simulink model "ATRIAS_vnmc"  (R2015a)
settings: Solver=ode45  StartTime=0.0  StopTime=60  FixedStep=1e-3  MinStep=1e-6  RelTol=1e-3  AbsTol=1e-4
values from neighbouring files (symbols this model uses):
  initial_boom_yaw = initial_boom_yaw + delta_yaw0    [run_model.m]
  max_floor_diff = cost_fun_opts.max_floor_diff    [opt_cmaes.m]    (also in run_model.m; set_all_params_simple.m = 0)
  noise_on_off = cost_fun_opts.noise_on_off    [opt_cmaes.m]    (also in run_model.m; set_all_params_simple.m = 0)
  noise_seed = cost_fun_opts.noise_seed    [opt_cmaes.m]    (also in run_model.m; set_all_params_simple.m = 1)
  noise_variance = cost_fun_opts.noise_variance    [opt_cmaes.m]    (also in run_model.m; set_all_params_simple.m = 0.000174532925199)
  SEA_swing_ctrl_on_off = cost_fun_opts.SEA_swing_ctrl_on_off    [opt_cmaes.m]    (also in run_model.m; set_all_params_simple.m = 0)
  sim_t = simout.twalk    [run_model.m]
  steady_dist = cost_fun_opts.steady_dist    [opt_cmaes.m]    (also in run_model.m; set_all_params_simple.m = 10)
  ts_anim = 0.0333    [run_model.m]
undefined symbols (not defined in the file or in its folder): A1_notch_f1, A2_notch_f1, A_lpf_dtau, A_lpf_velocity, B1_lpf_dtau, B1_lpf_velocity, B1_notch_f1, B2_lpf_dtau, B2_lpf_velocity, B2_notch_f1, b_hmotor, b_leg_spring, b_rotor, base_color_d, boom_color_d, boom_mount_to_center_diagonal, breakaway_friction, c, c_jointstop, com_height_offset, contactThr, coulomb_friction, CtrlPar_theta0, D12_S, D12_T, d_com, ddx_max, ddy_max, delta_phi_max, delta_phi_max_buffer, delta_phi_max_dropoff, delta_phi_min, des_forward_velocity, DS_width, dtau_des_max, dtheta0_vmc, dx0_vmc, dy_max, eref, fblink_color_d, fcut_acceleration, floor_color_d, floor_tile_width, floor_zero_height, FmaxBFSH, FmaxGLU, FmaxHAM, FmaxHFL, FmaxRF, FmaxVAS, FPCtrlPar, friction_linear_zone, g, gain_nodes_sea_torque, gamma_stance_thr, gamma_swing_thr, hip_height, HIP_MTR_MAX_CONT_TORQUE, HIP_MTR_MAX_TORQUE, hshaft_color_d ... (+236)
libraries: sm_lib x280, nesl_utility x174, simulink x114, simulink_extras x58, fl_lib x16, mblibv1 x2, dspswit3 x2
(part 7 of 23)

== system ATRIAS_vnmc/control/Add Limit Avoidance PD Torques/dtau_des ==
  x : Inport
  Gain1 : Gain  Gain=1/sample_time
  difference : simulink/Discrete/Difference  ICPrevInput=0.0  InputProcessing=Inherited  OutMin=[]  OutMax=[]  OutDataType=fixdt(1, 16)  OutScaling=2^-10  DoSatur=off
  two_pole_filter : DiscreteTransferFcn  Numerator=[A_lpf_dtau 0 0]  Denominator=[1 B1_lpf_dtau B2_lpf_dtau]  SampleTime=sample_time
  dx/dt : Outport
  wires:
  two_pole_filter/1 -> dx/dt/1
  x/1 -> Gain1/1
  difference/1 -> two_pole_filter/1
  Gain1/1 -> difference/1

== system ATRIAS_vnmc/control/Add Limit Avoidance PD Torques/mechanical limit avoidance ==
  tau_des [Nm]x4 : Inport
  PD Joint Limit : Subsystem
  Product : Product
  Sum : Sum  Inputs=++|
  tau_des + pd [Nm]x4 : Outport
  wires:
  tau_des [Nm]x4/1 -> Product/2
  PD Joint Limit/1(tau_pd [Nm]x4) -> Sum/1
  Sum/1 -> tau_des + pd [Nm]x4/1
  PD Joint Limit/2(des_trq_scale x4) -> Product/1
  Product/1 -> Sum/2

== system ATRIAS_vnmc/control/Export Results/Contact and GRFs ==
  note: BASED ON Leg Load
  note: BASED ON Foot Height
  Data Type Conversion{1..3,12} (4 alike) : DataTypeConversion  OutDataTypeStr=double
  Mux1 : Mux  Inputs=2
  Mux2 : Mux  Inputs=2
  Mux3 : Mux  Inputs=3
  Mux4 : Mux  Inputs=2
  10 : Outport
  wires:
  [RHeelCont] -> Data Type Conversion12/1
  [LHeelCont] -> Data Type Conversion1/1
  Mux3/1 -> 10/1
  Mux1/1 -> Mux3/1  "2"
  Data Type Conversion12/1 -> Mux1/1
  Data Type Conversion1/1 -> Mux1/2
  [RHeel_GRF] -> Mux2/1
  Mux2/1 -> Mux3/3  "2x3"
  [LHeel_GRF] -> Mux2/2
  [RFootCnt] -> Data Type Conversion3/1
  [LFootCnt] -> Data Type Conversion2/1
  Data Type Conversion3/1 -> Mux4/1
  Data Type Conversion2/1 -> Mux4/2
  Mux4/1 -> Mux3/2  "2"

== system ATRIAS_vnmc/control/Export Results/Segment Kinematics (position, orientation) ==
  Mux1 : Mux  Inputs=14
  Mux2 : Mux  Inputs=14
  Mux6 : Mux  Inputs=2
  98 : Outport
  wires:
  [xyzBoomBase] -> Mux1/1
  [xyzYawShaft] -> Mux1/2
  [xyzBoom] -> Mux1/3
  [xyzTorso] -> Mux1/4
  [RxyzHipShaft] -> Mux1/5
  [RxyzThigh] -> Mux1/6
  [RxyzShin] -> Mux1/7
  [RxyzLowerLeg] -> Mux1/8
  [RxyzFBlink] -> Mux1/9
  [LxyzLowerLeg] -> Mux1/13
  [LxyzFBlink] -> Mux1/14
  [LxyzHipShaft] -> Mux1/10
  [LxyzThigh] -> Mux1/11
  [LxyzShin] -> Mux1/12
  Mux1/1 -> Mux6/1  "position 42 = 14x3"
  [QBoomBase] -> Mux2/1
  [QYawShaft] -> Mux2/2
  [QBoom] -> Mux2/3
  [QTorso] -> Mux2/4
  [RQHipShaft] -> Mux2/5
  [RQThigh] -> Mux2/6
  [RQShin] -> Mux2/7
  [RQLowerLeg] -> Mux2/8
  [RQFBlink] -> Mux2/9
  [LQHipShaft] -> Mux2/10
  [LQThigh] -> Mux2/11
  [LQShin] -> Mux2/12
  [LQLowerLeg] -> Mux2/13
  [LQFBlink] -> Mux2/14
  Mux2/1 -> Mux6/2  "orientaion 56 = 14x4"
  Mux6/1 -> 98/1

== system ATRIAS_vnmc/control/Export Results/alpha targets ==
  Mux19 : Mux  Inputs=2
  2 : Outport
  wires:
  Mux19/1 -> 2/1
  [Ralpha_tgt] -> Mux19/1
  [Lalpha_tgt] -> Mux19/2

== system ATRIAS_vnmc/control/Export Results/track yaw ==
  xz : Inport
  Abs : Abs
  Compare To Constant : simulink/Logic and Bit Operations/Compare To Constant  relop=>  const=pi  OutDataTypeStr=boolean
  Gain : Gain  Gain=180/pi
  Gain1 : Gain  Gain=180/pi
  Gain2 : Gain  Gain=180/pi
  Memory : Memory
  Scope : Scope  NumInputPorts=4
      settings: YMin=-5~-5~-5~-5  YMax=5~5~5~5
  Sign : Signum
  Sum1 : Sum  Inputs=++|
  Sum2 : Sum  Inputs=|-+
  n*2*pi : Subsystem  TreatAsAtomicUnit=on
  "xz_to_yaw ([0, 2*pi])" : Fcn  Expr=atan2(u(1),-u(2)) +2*pi*(atan2(u(1),-u(2))<0)
  yaw : Outport
  wires:
  Sign/1 -> n*2*pi/2(sign)
  xz/1 -> "xz_to_yaw ([0, 2*pi])"/1
  "xz_to_yaw ([0, 2*pi])"/1 -> Memory/1, Gain1/1, Sum1/2, Sum2/2
  n*2*pi/1(n*2*pi) -> Gain/1, n*2*pi/1((n-1)*2*pi), Sum1/1
  Sum2/1 -> Sign/1, Abs/1
  Abs/1 -> Gain2/1, Compare To Constant/1
  Memory/1 -> Sum2/1
  Compare To Constant/1 -> Scope/3, n*2*pi/Trigger
  Sum1/1 -> yaw/1
  Gain/1 -> Scope/1
  Gain1/1 -> Scope/2
  Gain2/1 -> Scope/4

== system ATRIAS_vnmc/control/Monitor Simulation/Check Ground Penetration ==
  xyz : Inport
  Ground H : Interpolation_n-D  NumberOfTableDimensions=1  Table=v_plateH
      settings: InputPortMap=u0,u1
  Prelookup : PreLookup  BreakpointsData=v_plateYaw  ExtrapMethod=Linear
  Relational Operator : RelationalOperator  Operator=<=  OutDataTypeStr=boolean
  Selector1 : Selector  InputPortWidth=3  Indices=[1 3]
  Selector2 : Selector  InputPortWidth=3  Indices=2
  track yaw : Subsystem
  Below Ground : Outport
  wires:
  Prelookup/2 -> Ground H/2
  track yaw/1(yaw) -> Prelookup/1
  Prelookup/1 -> Ground H/1
  Selector1/1 -> track yaw/1(xz)
  Relational Operator/1 -> Below Ground/1
  Selector2/1 -> Relational Operator/1
  xyz/1 -> Selector1/1, Selector2/1
  Ground H/1 -> Relational Operator/2

== system ATRIAS_vnmc/control/Monitor Simulation/Check Ground Penetration1 ==
  xyz : Inport
  Ground H : Interpolation_n-D  NumberOfTableDimensions=1  Table=v_plateH
      settings: InputPortMap=u0,u1
  Prelookup : PreLookup  BreakpointsData=v_plateYaw  ExtrapMethod=Linear
  Relational Operator : RelationalOperator  Operator=<=  OutDataTypeStr=boolean
  Selector1 : Selector  InputPortWidth=3  Indices=[1 3]
  Selector2 : Selector  InputPortWidth=3  Indices=2
  track yaw : Subsystem
  Below Ground : Outport
  wires:
  Prelookup/2 -> Ground H/2
  track yaw/1(yaw) -> Prelookup/1
  Prelookup/1 -> Ground H/1
  Selector1/1 -> track yaw/1(xz)
  Relational Operator/1 -> Below Ground/1
  Selector2/1 -> Relational Operator/1
  xyz/1 -> Selector1/1, Selector2/1
  Ground H/1 -> Relational Operator/2

== system ATRIAS_vnmc/control/Monitor Simulation/Check Ground Penetration2 ==
  xyz : Inport
  Ground H : Interpolation_n-D  NumberOfTableDimensions=1  Table=v_plateH
      settings: InputPortMap=u0,u1
  Prelookup : PreLookup  BreakpointsData=v_plateYaw  ExtrapMethod=Linear
  Relational Operator : RelationalOperator  Operator=<=  OutDataTypeStr=boolean
  Selector1 : Selector  InputPortWidth=3  Indices=[1 3]
  Selector2 : Selector  InputPortWidth=3  Indices=2
  track yaw : Subsystem
  Below Ground : Outport
  wires:
  Prelookup/2 -> Ground H/2
  track yaw/1(yaw) -> Prelookup/1
  Prelookup/1 -> Ground H/1
  Selector1/1 -> track yaw/1(xz)
  Relational Operator/1 -> Below Ground/1
  Selector2/1 -> Relational Operator/1
  xyz/1 -> Selector1/1, Selector2/1
  Ground H/1 -> Relational Operator/2

== system ATRIAS_vnmc/control/Monitor Simulation/Check Ground Penetration3 ==
  xyz : Inport
  Ground H : Interpolation_n-D  NumberOfTableDimensions=1  Table=v_plateH
      settings: InputPortMap=u0,u1
  Prelookup : PreLookup  BreakpointsData=v_plateYaw  ExtrapMethod=Linear
  Relational Operator : RelationalOperator  Operator=<=  OutDataTypeStr=boolean
  Selector1 : Selector  InputPortWidth=3  Indices=[1 3]
  Selector2 : Selector  InputPortWidth=3  Indices=2
  track yaw : Subsystem
  Below Ground : Outport
  wires:
  Prelookup/2 -> Ground H/2
  track yaw/1(yaw) -> Prelookup/1
  Prelookup/1 -> Ground H/1
  Selector1/1 -> track yaw/1(xz)
  Relational Operator/1 -> Below Ground/1
  Selector2/1 -> Relational Operator/1
  xyz/1 -> Selector1/1, Selector2/1
  Ground H/1 -> Relational Operator/2

== system ATRIAS_vnmc/control/Monitor Simulation/Step Length History ==
  footstrike : Inport
  Lx_Heel : Inport  Port=2
  LHeelCont : Inport  Port=3
  RHeelCont : Inport  Port=4
  RxHeel : Inport  Port=5
  Measure Step Length : Subsystem  TreatAsAtomicUnit=on
  Memory1 : Memory
  Queue1 : Subsystem
  x_footstrike : Subsystem
  step length hist : Outport
  wires:
  Lx_Heel/1 -> x_footstrike/2(x_LFoot [m])
  x_footstrike/1(x_footstrike [m]) -> Measure Step Length/2(x_heelstrike [m]), Memory1/1
  LHeelCont/1 -> x_footstrike/3(LHeel Contact [1/0])
  Memory1/1 -> Measure Step Length/1(x_heelstrike_prev [m])
  Measure Step Length/1(Step Length [m]) -> Queue1/2(stepLength0 [m])
  Queue1/1(footLengthHist [m,m,m,m,m,m,m]) -> step length hist/1
  RxHeel/1 -> x_footstrike/5(x_RFoot [m])
  RHeelCont/1 -> x_footstrike/4(RHeel Contact [1/0])
  footstrike/1 -> Queue1/1(footStrike [1/0]), Measure Step Length/Trigger, x_footstrike/1(Footstrike [1/0])

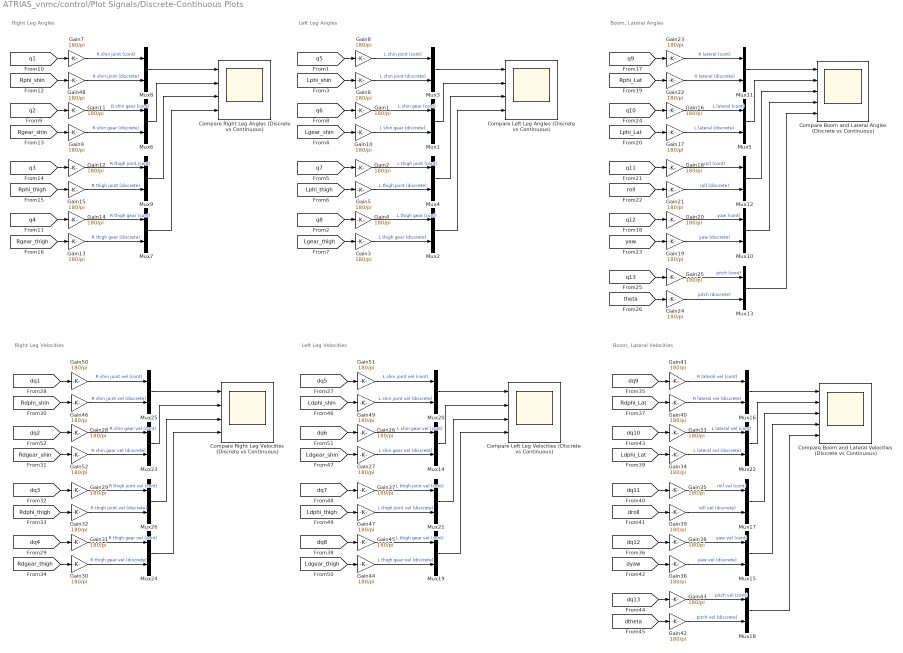
== system ATRIAS_vnmc/control/Plot Signals/Discrete-Continuous Plots ==
  note: Right Leg Angles
  note: Left Leg Angles
  note: Boom, Lateral Angles
  note: Right Leg Velocities
  note: Left Leg Velocities
  note: Boom, Lateral Velocities
  Compare Boom and Lateral Angles (Discrete vs Continuous) : Scope  NumInputPorts=5
      settings: ShowLegends=on  TimeRange=0.895  YMin=152~225.5~132~205.5~-5  YMax=154.5~228~134.5~208~5  SaveName=ScopeData12
  Compare Boom and Lateral Velocities (Discrete vs Continuous) : Scope  NumInputPorts=5
      settings: ShowLegends=on  TimeRange=0.895  YMin=152~225.5~132~205.5~-5  YMax=154.5~228~134.5~208~5  SaveName=ScopeData13
  Compare Left Leg Angles (Discrete vs Continuous) : Scope  NumInputPorts=4
      settings: ShowLegends=on  TimeRange=0.895  YMin=152~225.5~132~205.5  YMax=154.5~228~134.5~208  SaveName=ScopeData11
  Compare Left Leg Velocities (Discrete vs Continuous) : Scope  NumInputPorts=4
      settings: ShowLegends=on  TimeRange=0.895  YMin=152~225.5~132~205.5  YMax=154.5~228~134.5~208  SaveName=ScopeData14
  Compare Right Leg Angles (Discrete vs Continuous) : Scope  NumInputPorts=4
      settings: ShowLegends=on  TimeRange=0.895  YMin=152~225.5~132~205.5  YMax=154.5~228~134.5~208  SaveName=ScopeData8
  Compare Right Leg Velocities (Discrete vs Continuous) : Scope  NumInputPorts=4
      settings: ShowLegends=on  TimeRange=0.895  YMin=152~225.5~132~205.5  YMax=154.5~228~134.5~208  SaveName=ScopeData15
  Gain{1..52} (52 alike) : Gain  Gain=180/pi
  Mux{1..26} (26 alike) : Mux  Inputs=2
  wires:
  [Rphi_thigh] -> Gain15/1
  [q4] -> Gain14/1
  [q3] -> Gain12/1
  Gain14/1 -> Mux7/1  "R thigh gear (cont)"
  Gain12/1 -> Mux9/1  "R thigh joint (cont)"
  Gain15/1 -> Mux9/2  "R thigh joint (discrete)"
  Mux7/1 -> Compare Right Leg Angles (Discrete vs Continuous)/4
  Gain13/1 -> Mux7/2  "R thigh gear (discrete)"
  Mux9/1 -> Compare Right Leg Angles (Discrete vs Continuous)/3
  [Rgear_thigh] -> Gain13/1
  [Rphi_shin] -> Gain48/1
  [q2] -> Gain11/1
  [q1] -> Gain7/1
  Gain11/1 -> Mux6/1  "R shin gear (cont)"
  Gain7/1 -> Mux8/1  "R shin joint (cont)"
  Gain48/1 -> Mux8/2  "R shin joint (discrete)"
  Mux6/1 -> Compare Right Leg Angles (Discrete vs Continuous)/2
  Gain9/1 -> Mux6/2  "R shin gear (discrete)"
  Mux8/1 -> Compare Right Leg Angles (Discrete vs Continuous)/1
  [Rgear_shin] -> Gain9/1
  [Lphi_thigh] -> Gain5/1
  [q8] -> Gain4/1
  [q7] -> Gain2/1
  Gain4/1 -> Mux2/1  "L thigh gear (cont)"
  Gain2/1 -> Mux4/1  "L thigh joint (cont)"
  Gain5/1 -> Mux4/2  "L thigh joint (discrete)"
  Mux2/1 -> Compare Left Leg Angles (Discrete vs Continuous)/4
  Gain3/1 -> Mux2/2  "L thigh gear (discrete)"
  Mux4/1 -> Compare Left Leg Angles (Discrete vs Continuous)/3
  [Lgear_thigh] -> Gain3/1
  [Lphi_shin] -> Gain6/1
  [q6] -> Gain1/1
  [q5] -> Gain8/1
  Gain1/1 -> Mux1/1  "L shin gear (cont)"
  Gain8/1 -> Mux3/1  "L shin joint (cont)"
  Gain6/1 -> Mux3/2  "L shin joint (discrete)"
  Mux1/1 -> Compare Left Leg Angles (Discrete vs Continuous)/2
  Gain10/1 -> Mux1/2  "L shin gear (discrete)"
  Mux3/1 -> Compare Left Leg Angles (Discrete vs Continuous)/1
  [Lgear_shin] -> Gain10/1
  [roll] -> Gain21/1
  [q12] -> Gain20/1
  [q11] -> Gain18/1
  Gain20/1 -> Mux10/1  "yaw (cont)"
  Gain18/1 -> Mux12/1  "roll (cont)"
  Gain21/1 -> Mux12/2  "roll (discrete)"
  Mux10/1 -> Compare Boom and Lateral Angles (Discrete vs Continuous)/4
  Gain19/1 -> Mux10/2  "yaw (discrete)"
  Mux12/1 -> Compare Boom and Lateral Angles (Discrete vs Continuous)/3
  [yaw] -> Gain19/1
  [Rphi_Lat] -> Gain22/1
  [q10] -> Gain16/1
  [q9] -> Gain23/1
  Gain16/1 -> Mux5/1  "L lateral (cont)"
  Gain23/1 -> Mux11/1  "R lateral (cont)"
  Gain22/1 -> Mux11/2  "R lateral (discrete)"
  Mux5/1 -> Compare Boom and Lateral Angles (Discrete vs Continuous)/2
  Gain17/1 -> Mux5/2  "L lateral (discrete)"
  Mux11/1 -> Compare Boom and Lateral Angles (Discrete vs Continuous)/1
  [Lphi_Lat] -> Gain17/1
  [q13] -> Gain25/1
  Gain25/1 -> Mux13/1  "pitch (cont)"
  Mux13/1 -> Compare Boom and Lateral Angles (Discrete vs Continuous)/5
  Gain24/1 -> Mux13/2  "pitch (discrete)"
  [theta] -> Gain24/1
  [Rdphi_thigh] -> Gain32/1
  [dq4] -> Gain31/1
  [dq3] -> Gain29/1
  Gain31/1 -> Mux24/1  "R thigh gear vel (cont)"
  Gain29/1 -> Mux26/1  "R thigh joint vel (cont)"
  Gain32/1 -> Mux26/2  "R thigh joint vel (discrete)"
  Mux24/1 -> Compare Right Leg Velocities (Discrete vs Continuous)/4
  Gain30/1 -> Mux24/2  "R thigh gear vel (discrete)"
  Mux26/1 -> Compare Right Leg Velocities (Discrete vs Continuous)/3
  [Rdgear_thigh] -> Gain30/1
  [Rdphi_shin] -> Gain46/1
  [dq2] -> Gain28/1
  [dq1] -> Gain50/1
  Gain28/1 -> Mux23/1  "R shin gear vel (cont)"
  Gain50/1 -> Mux25/1  "R shin joint vel (cont)"
  Gain46/1 -> Mux25/2  "R shin joint vel (discrete)"
  Mux23/1 -> Compare Right Leg Velocities (Discrete vs Continuous)/2
  Gain52/1 -> Mux23/2  "R shin gear vel (discrete)"
  Mux25/1 -> Compare Right Leg Velocities (Discrete vs Continuous)/1
  [Rdgear_shin] -> Gain52/1
  [Ldphi_thigh] -> Gain47/1
  [dq8] -> Gain45/1
  [dq7] -> Gain37/1
  Gain45/1 -> Mux19/1  "L thigh gear vel (cont)"
  Gain37/1 -> Mux21/1  "L thigh joint vel (cont)"
  Gain47/1 -> Mux21/2  "L thigh joint vel (discrete)"
  Mux19/1 -> Compare Left Leg Velocities (Discrete vs Continuous)/4
  Gain44/1 -> Mux19/2  "L thigh gear vel (discrete)"
  Mux21/1 -> Compare Left Leg Velocities (Discrete vs Continuous)/3
  [Ldgear_thigh] -> Gain44/1
  [Ldphi_shin] -> Gain49/1
  [dq6] -> Gain26/1
  [dq5] -> Gain51/1
  Gain26/1 -> Mux14/1  "L shin gear vel (cont)"
  Gain51/1 -> Mux20/1  "L shin joint vel (cont)"
  Gain49/1 -> Mux20/2  "L shin joint vel (discrete)"
  Mux14/1 -> Compare Left Leg Velocities (Discrete vs Continuous)/2
  Gain27/1 -> Mux14/2  "L shin gear vel (discrete)"
  Mux20/1 -> Compare Left Leg Velocities (Discrete vs Continuous)/1
  [Ldgear_shin] -> Gain27/1
  [droll] -> Gain39/1
  [dq12] -> Gain38/1
  [dq11] -> Gain35/1
  Gain38/1 -> Mux15/1  "yaw vel (cont)"
  Gain35/1 -> Mux17/1  "roll vel (cont)"
  Gain39/1 -> Mux17/2  "roll vel (discrete)"
  Mux15/1 -> Compare Boom and Lateral Velocities (Discrete vs Continuous)/4
  Gain36/1 -> Mux15/2  "yaw vel (discrete)"
  Mux17/1 -> Compare Boom and Lateral Velocities (Discrete vs Continuous)/3
  [dyaw] -> Gain36/1
  [Rdphi_Lat] -> Gain40/1
  [dq10] -> Gain33/1
  [dq9] -> Gain41/1
  Gain33/1 -> Mux22/1  "L lateral vel (cont)"
  Gain41/1 -> Mux16/1  "R lateral vel (cont)"
  Gain40/1 -> Mux16/2  "R lateral vel (discrete)"
  Mux22/1 -> Compare Boom and Lateral Velocities (Discrete vs Continuous)/2
  Gain34/1 -> Mux22/2  "L lateral vel (discrete)"
  Mux16/1 -> Compare Boom and Lateral Velocities (Discrete vs Continuous)/1
  [Ldphi_Lat] -> Gain34/1
  [dq13] -> Gain43/1
  Gain43/1 -> Mux18/1  "pitch vel (cont)"
  Mux18/1 -> Compare Boom and Lateral Velocities (Discrete vs Continuous)/5
  Gain42/1 -> Mux18/2  "pitch vel (discrete)"
  [dtheta] -> Gain42/1

== system ATRIAS_vnmc/control/Plot Signals/GRFs, leg load, contact ==
  Add : Sum
  Constant : Constant  Value=contactThr
  Constant1 : Constant  Value=releaseThr
  Data Type Conversion : DataTypeConversion  OutDataTypeStr=double
  Data Type Conversion1 : DataTypeConversion  OutDataTypeStr=double
  Demux : Demux
  "GRFs, Leg Load, Contact" : Scope  NumInputPorts=4
      settings: ShowLegends=on  TimeRange=0.4076343628585122  YMin=0~-1~-1400~0  YMax=2.5~1.5~0~2000  SaveName=ScopeData28
  Mux1 : Mux
  Mux2 : Mux  Inputs=2
  Mux23 : Mux  Inputs=2
  Mux3 : Mux
  Mux58 : Mux
  Selector39 : Selector  InputPortWidth=3
  Selector41 : Selector  InputPortWidth=3  Indices=2
  Selector43 : Selector  InputPortWidth=3
  Selector45 : Selector  InputPortWidth=3  Indices=2
  plot offset : Constant  Value=[0.5 -0.9 0.4 -1]
  wires:
  Selector39/1 -> Mux2/1  "LGRF_Heel_x"
  [RLLoad] -> Mux58/2  "R Leg Load [bw]"
  [LLLoad] -> Mux58/1  "L Leg Load [bw]"
  Mux58/1 -> "GRFs, Leg Load, Contact"/1
  Mux23/1 -> "GRFs, Leg Load, Contact"/4
  Selector41/1 -> Mux23/1  "LGRF_Heel_y"
  [RHeel_GRF] -> Selector45/1, Selector43/1
  Selector43/1 -> Mux2/2  "RGRF_Heel_x"
  Selector45/1 -> Mux23/2  "RGRF_Heel_y"
  [LHeel_GRF] -> Selector39/1, Selector41/1
  Mux2/1 -> "GRFs, Leg Load, Contact"/3
  Constant/1 -> Mux58/3  "contact threshold"
  Constant1/1 -> Mux58/4  "release threshold"
  [LFootCnt] -> Mux3/2  "L Contact Detection"
  [RFootCnt] -> Mux3/1  "R Contact Detection"
  Mux1/1 -> "GRFs, Leg Load, Contact"/2
  [RHeelCont] -> Data Type Conversion/1
  [LHeelCont] -> Data Type Conversion1/1
  Mux3/1 -> Add/1
  plot offset/1 -> Add/2
  Demux/1 -> Mux1/1  "R Contact Detection"
  Demux/2 -> Mux1/2  "L Contact Detection"
  Demux/3 -> Mux1/3  "R Contact"
  Demux/4 -> Mux1/4  "L Contact"
  Add/1 -> Demux/1
  Data Type Conversion/1 -> Mux3/3
  Data Type Conversion1/1 -> Mux3/4

== system ATRIAS_vnmc/control/Plot Signals/Markers ==
  Demux : Demux  Commented=on  Outputs=3
  Demux1 : Demux  Commented=on  Outputs=3
  Demux{2..5} (4 alike) : Demux  Commented=on
  From141 : From  Commented=on  GotoTag=xyzHAT
  From142 : From  Commented=on  GotoTag=xyzHead
  From143 : From  Commented=on  GotoTag=xyzHips
  From147 : From  Commented=on  GotoTag=LxyzHeel  TagVisibility=global
  From148 : From  Commented=on  GotoTag=LxyzShank
  From149 : From  Commented=on  GotoTag=LxyzLowerThigh
  From150 : From  Commented=on  GotoTag=LxyzUpperThigh
  From153 : From  Commented=on  GotoTag=RxyzHeel  TagVisibility=global
  From154 : From  Commented=on  GotoTag=RxyzShank
  From155 : From  Commented=on  GotoTag=RxyzLowerThigh
  From156 : From  Commented=on  GotoTag=RxyzUpperThigh
  Marker Positions : Scope  Commented=on  NumInputPorts=6
      settings: ShowLegends=on  TimeRange=60  YMin=60~-2.5e+09~-5e+09~-5~-5~-5  YMax=140~2.5e+10~4e+09~5~5~5  SaveName=ScopeData6
  Mux33 : Mux  Commented=on  Inputs=3
  Mux{34..35,38..41} (6 alike) : Mux  Commented=on
  Mux36 : Mux  Commented=on  Inputs=3
  Mux37 : Mux  Commented=on  Inputs=3
  xLeft : Selector  Commented=on  InputPortWidth=12  Indices=[1 4 7 10]
  xRight : Selector  Commented=on  InputPortWidth=12  Indices=[1 4 7 10]
  xtorso : Selector  Commented=on  InputPortWidth=9  Indices=[1 4 7]
  yLeft : Selector  Commented=on  InputPortWidth=12  Indices=[2 5 8 11]
  yRight : Selector  Commented=on  InputPortWidth=12  Indices=[2 5 8 11]
  ytorso : Selector  Commented=on  InputPortWidth=9  Indices=[2 5 8]
  wires:
  Mux36/1 -> Marker Positions/1
  Demux/2 -> Mux36/2  "xCOM"
  Mux34/1 -> xLeft/1, yLeft/1
  Demux3/1 -> Mux39/1  "xLUpperThigh"
  Mux39/1 -> Marker Positions/3
  Demux3/2 -> Mux39/2  "xLLowerThigh"
  From154/1 -> Mux35/3
  From156/1 -> Mux35/1
  Demux/1 -> Mux36/1  "xHead"
  Mux40/1 -> Marker Positions/6
  From155/1 -> Mux35/2
  Demux5/2 -> Mux41/2  "xRLowerThigh"
  From143/1 -> Mux33/3
  xtorso/1 -> Demux/1
  Mux41/1 -> Marker Positions/5
  From141/1 -> Mux33/2
  yRight/1 -> Demux4/1
  From150/1 -> Mux34/1
  Demux5/4 -> Mux41/4  "xRHeel"
  From153/1 -> Mux35/4
  Demux5/1 -> Mux41/1  "xRUpperThigh"
  From148/1 -> Mux34/3
  Demux1/3 -> Mux37/3  "yHips"
  Mux37/1 -> Marker Positions/2
  Demux4/2 -> Mux40/2  "yRLowerThigh"
  ytorso/1 -> Demux1/1
  Mux33/1 -> ytorso/1, xtorso/1
  Demux2/3 -> Mux38/3  "yLShank"
  From149/1 -> Mux34/2
  From142/1 -> Mux33/1
  From147/1 -> Mux34/4
  Demux3/4 -> Mux39/4  "xLHeel"
  Demux2/4 -> Mux38/4  "yLHeel"
  xLeft/1 -> Demux3/1
  Demux1/2 -> Mux37/2  "yCOM"
  Demux3/3 -> Mux39/3  "xLShank"
  Demux/3 -> Mux36/3  "xHips"
  Mux35/1 -> yRight/1, xRight/1
  Demux1/1 -> Mux37/1  "yHead"
  Mux38/1 -> Marker Positions/4
  Demux2/1 -> Mux38/1  "yLUpperThigh"
  Demux2/2 -> Mux38/2  "yLLowerThigh"
  yLeft/1 -> Demux2/1
  Demux4/4 -> Mux40/4  "yRHeel"
  Demux5/3 -> Mux41/3  "xRShank"
  Demux4/3 -> Mux40/3  "yRShank"
  Demux4/1 -> Mux40/1  "yRUpperThigh"
  xRight/1 -> Demux5/1

== system ATRIAS_vnmc/control/Plot Signals/Robot Angles ==
  note: Left
  note: Right
  note: Joint/Gear
  Constant10 : Constant  Value=phi_shin_min+phi_shin_min_buffer
  Constant12 : Constant  Value=delta_phi_max-delta_phi_max_buffer
  Constant13 : Constant  Value=delta_phi_max
  Constant14 : Constant  Value=min_splay_angle
  Constant15 : Constant  Value=min_splay_angle+min_splay_buffer
  Constant16 : Constant  Value=phi_thigh_min+phi_thigh_min_buffer
  Constant17 : Constant  Value=phi_thigh_max-phi_thigh_max_buffer
  Constant18 : Constant  Value=phi_thigh_min
  Constant19 : Constant  Value=phi_thigh_max
  Constant2 : Constant  Value=phi_thigh_min
  Constant20 : Constant  Value=phi_shin_min+phi_shin_min_buffer
  Constant21 : Constant  Value=phi_shin_max-phi_shin_max_buffer
  Constant22 : Constant  Value=delta_phi_max-delta_phi_max_buffer
  Constant23 : Constant  Value=phi_shin_min
  Constant24 : Constant  Value=phi_shin_max
  Constant25 : Constant  Value=delta_phi_min
  Constant26 : Constant  Value=delta_phi_max
  Constant27 : Constant  Value=min_splay_angle
  Constant28 : Constant  Value=min_splay_angle+min_splay_buffer
  Constant29 : Constant  Value=phi_thigh_min+phi_thigh_min_buffer
  Constant30 : Constant  Value=phi_thigh_max-phi_thigh_max_buffer
  Constant5 : Constant  Value=phi_thigh_max
  Constant6 : Constant  Value=phi_shin_max-phi_shin_max_buffer
  Constant7 : Constant  Value=phi_shin_min
  Constant8 : Constant  Value=phi_shin_max
  Constant9 : Constant  Value=delta_phi_min
  Gain{1..14,16..47} (46 alike) : Gain  Gain=180/pi
  Joint/Gear : Scope  NumInputPorts=5
      settings: ShowLegends=on  TimeRange=0.895  YMin=152~225.5~132~205.5~-1  YMax=154.5~228~134.5~208~1  SaveName=ScopeData10
  L Robot Angles : Scope  NumInputPorts=3
      settings: ShowLegends=on  TimeRange=1.4  YMin=60~120~20  YMax=240~300~160  SaveName=ScopeData4
  Mux{1..4} (4 alike) : Mux  Inputs=2
  Mux5 : Mux
  Mux{88,90,96,98} (4 alike) : Mux  Inputs=6
  Mux89 : Mux  Inputs=7
  Mux97 : Mux  Inputs=7
  R Robot Angles : Scope  NumInputPorts=3
      settings: ShowLegends=on  TimeRange=0.895  YMin=60~120~20  YMax=240~300~160  SaveName=ScopeData2
  Sum : Sum  Inputs=|+-
  Sum1 : Sum  Inputs=|+-
  wires:
  Constant2/1 -> Gain23/1
  Gain28/1 -> Mux89/3  "absolute max splay angle"
  Constant9/1 -> Gain27/1
  Constant7/1 -> Gain25/1
  Mux90/1 -> L Robot Angles/1
  Gain25/1 -> Mux88/2  "min shin angle"
  Mux88/1 -> L Robot Angles/2
  Gain23/1 -> Mux90/2  "min thigh angle"
  Constant8/1 -> Gain26/1
  Gain24/1 -> Mux90/3  "max thigh angle"
  Gain26/1 -> Mux88/3  "max shin angle"
  Mux89/1 -> L Robot Angles/3
  Gain27/1 -> Mux89/7  "absolute min splay angle"
  Gain16/1 -> Mux90/1  "L thigh angle"
  Gain17/1 -> Mux88/1  "L shin angle"
  [Lphi_thigh] -> Gain16/1
  [Lphi_shin] -> Gain17/1
  Gain18/1 -> Mux89/1  "L Upper Splay  Angle"
  Constant5/1 -> Gain24/1
  Constant13/1 -> Gain28/1
  Gain19/1 -> Mux89/2  "min splay angle"
  Constant14/1 -> Gain19/1
  Constant15/1 -> Gain20/1
  Gain20/1 -> Mux89/4  "min splay buffer"
  Constant16/1 -> Gain21/1
  Gain21/1 -> Mux90/4  "min thigh buffer"
  Gain22/1 -> Mux90/5  "max thigh buffer"
  Constant17/1 -> Gain22/1
  Constant10/1 -> Gain29/1
  Gain29/1 -> Mux88/4  "min shin buffer"
  Constant6/1 -> Gain30/1
  Gain30/1 -> Mux88/5  "max shin buffer"
  Constant12/1 -> Gain31/1
  Gain31/1 -> Mux89/5  "max splay buffer"
  Constant18/1 -> Gain39/1
  Gain44/1 -> Mux97/3  "absolute max splay angle"
  Constant25/1 -> Gain43/1
  Constant23/1 -> Gain41/1
  Mux98/1 -> R Robot Angles/1
  Gain41/1 -> Mux96/2  "min shin angle"
  Mux96/1 -> R Robot Angles/2
  Gain39/1 -> Mux98/2  "min thigh angle"
  Constant24/1 -> Gain42/1
  Gain40/1 -> Mux98/3  "max thigh angle"
  Gain42/1 -> Mux96/3  "max shin angle"
  Mux97/1 -> R Robot Angles/3
  Gain43/1 -> Mux97/7  "absolute min splay angle"
  Gain32/1 -> Mux98/1  "R thigh angle"
  Gain33/1 -> Mux96/1  "R shin angle"
  [Rphi_thigh] -> Gain32/1
  [Rphi_shin] -> Gain33/1
  [Rsplay] -> Gain34/1
  Gain34/1 -> Mux97/1  "R Upper Splay  Angle"
  Constant19/1 -> Gain40/1
  Constant26/1 -> Gain44/1
  Gain35/1 -> Mux97/2  "min splay angle"
  Constant27/1 -> Gain35/1
  Constant28/1 -> Gain36/1
  Gain36/1 -> Mux97/4  "min splay buffer"
  Constant29/1 -> Gain37/1
  Gain37/1 -> Mux98/4  "min thigh buffer"
  Gain38/1 -> Mux98/5  "max thigh buffer"
  Constant30/1 -> Gain38/1
  Constant20/1 -> Gain45/1
  Gain45/1 -> Mux96/4  "min shin buffer"
  Constant21/1 -> Gain46/1
  Gain46/1 -> Mux96/5  "max shin buffer"
  Constant22/1 -> Gain47/1
  Gain47/1 -> Mux97/5  "max splay buffer"
  [Lsplay] -> Gain18/1
  [Rgear_shin] -> Gain10/1
  Mux3/1 -> Joint/Gear/1
  Gain10/1 -> Mux1/2  "R gear angle"
  Mux1/1 -> Joint/Gear/2
  Gain8/1 -> Mux3/2  "R gear angle"
  Gain1/1 -> Mux3/1  "R thigh angle"
  Gain2/1 -> Mux1/1  "R shin angle"
  [Rphi_thigh] -> Gain1/1
  [Rphi_shin] -> Gain2/1
  [Rgear_thigh] -> Gain8/1
  [Lgear_shin] -> Gain4/1
  Mux4/1 -> Joint/Gear/3
  Gain4/1 -> Mux2/2  "L gear angle"
  Mux2/1 -> Joint/Gear/4
  Gain6/1 -> Mux4/2  "L gear angle"
  Gain3/1 -> Mux4/1  "L thigh angle"
  Gain5/1 -> Mux2/1  "L shin angle"
  [Lphi_thigh] -> Gain3/1
  [Lphi_shin] -> Gain5/1
  [Lgear_thigh] -> Gain6/1
  [RtauB] -> Mux5/1  "R tau meas back"
  [RtauF] -> Mux5/2  "R tau meas front"
  [LtauF] -> Mux5/3  "L tau meas back"
  [LtauB] -> Mux5/4  "L tau meas front"
  Mux5/1 -> Joint/Gear/5
  Gain7/1 -> Mux90/6  "L thigh gear"
  [Lgear_thigh] -> Gain7/1
  Gain9/1 -> Mux88/6  "L shin gear"
  [Lgear_shin] -> Gain9/1
  Gain11/1 -> Mux89/6  "L splay gear"
  [Lgear_shin] -> Sum/1
  [Lgear_thigh] -> Sum/2
  Sum/1 -> Gain11/1
  Gain12/1 -> Mux97/6  "L splay gear"
  [Rgear_shin] -> Sum1/1
  [Rgear_thigh] -> Sum1/2
  Sum1/1 -> Gain12/1
  Gain13/1 -> Mux96/6  "L shin gear"
  [Rgear_shin] -> Gain13/1
  Gain14/1 -> Mux98/6  "L thigh gear"
  [Rgear_thigh] -> Gain14/1

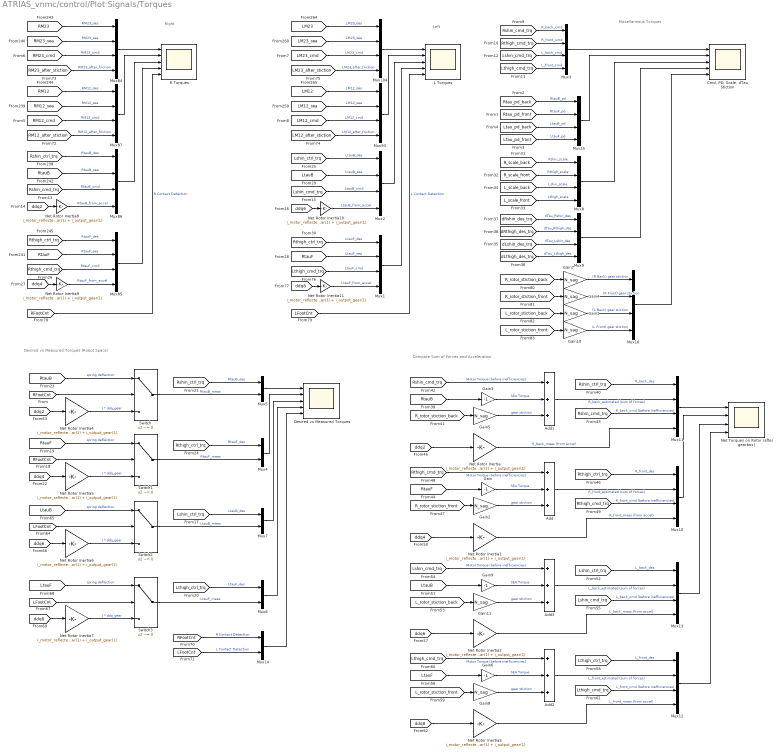
== system ATRIAS_vnmc/control/Plot Signals/Torques ==
  note: Right
  note: Left
  note: Desired vs Measured Torques (Robot Space)
  note: Compare Sum of Forces and Acceleration
  note: Miscellaneous Torques
  Add{,1..3} (4 alike) : Sum  Inputs=+++
  "Cmd, PD, Scale, dTau, Stiction" : Scope  NumInputPorts=5
      settings: ShowLegends=on  TimeRange=1.4  YMin=-300~-3500~-5~-5~-5  YMax=400~1000~5~5~5  SaveName=ScopeData9
  Desired vs Measured Torques : Scope  NumInputPorts=5
      settings: ShowLegends=on  TimeRange=0.748  YMin=220~-150~-40~-30~-5  YMax=360~-80~30~10~5  SaveName=ScopeData20
  Gain{,3,6,9} (4 alike) : Gain  Gain=-1
  Gain{1..2,4..5,7..8,10..11} (8 alike) : Gain  Gain=N_sag
  L Torques : Scope  NumInputPorts=5
      settings: ShowLegends=on  TimeRange=0.748  YMin=-600~-1000~-400~-600~-5  YMax=600~1000~800~200~5  SaveName=ScopeData7
  Mux{1..3,8..13,15..16,84..87,93,104} (17 alike) : Mux
  Mux{4..7,14} (5 alike) : Mux  Inputs=2
  Net Rotor Inertia{,1..11} (12 alike) : Gain  Gain=i_motor_reflected(1) + i_virtual_gear(1) + i_output_gear(1)
  Net Torques on Rotor (after gearbox) : Scope  NumInputPorts=4
      settings: ShowLegends=on  TimeRange=0.748  YMin=220~-150~-40~-30  YMax=360~-80~30~10  SaveName=ScopeData21
  R Torques : Scope  NumInputPorts=5
      settings: ShowLegends=on  TimeRange=0.748  YMin=-400~-800~-400~-300~-5  YMax=400~600~600~200~5  SaveName=ScopeData3
  Switch{,1..3} (4 alike) : Switch  Criteria=u2 ~= 0
  wires:
  [LM12] -> Mux93/1  "LM12_des"
  [LM23] -> Mux104/1  "LM23_des"
  [LM12_sea] -> Mux93/2  "LM12_sea"
  [LM23_sea] -> Mux104/2  "LM23_sea"
  [Rshin_ctrl_trq] -> Mux86/1  "RtauB_des"
  [RtauF] -> Mux85/2  "RtauF_sea"
  [RtauB] -> Mux86/2  "RtauB_sea"
  [RM12] -> Mux87/1  "RM12_des"
  [RM23] -> Mux84/1  "RM23_des"
  [RM12_sea] -> Mux87/2  "RM12_sea"
  [RM23_sea] -> Mux84/2  "RM23_sea"
  [RM12_cmd] -> Mux87/3  "RM12_cmd"
  [RM23_cmd] -> Mux84/3  "RM23_cmd"
  [LM23_cmd] -> Mux104/3  "LM23_cmd"
  [LM12_cmd] -> Mux93/3  "LM12_cmd"
  [Rthigh_ctrl_trq] -> Mux4/1  "RtauF_des"
  [Rshin_ctrl_trq] -> Mux5/1  "RtauB_des"
  Switch1/1 -> Mux4/2  "RtauF_meas"
  Switch/1 -> Mux5/2  "RtauB_meas"
  [Lthigh_ctrl_trq] -> Mux6/1  "LtauF_des"
  [Lshin_ctrl_trq] -> Mux7/1  "LtauB_des"
  Switch3/1 -> Mux6/2  "LtauF_meas"
  Switch2/1 -> Mux7/2  "LtauB_meas"
  [Rthigh_ctrl_trq] -> Mux85/1  "RtauF_des"
  [Rthigh_ctrl_trq] -> Mux10/1  "R_front_des"
  [RtauF] -> Gain/1
  [R_rotor_stiction_front] -> Gain2/1
  Gain2/1 -> Add/3  "gear stiction"
  Gain/1 -> Add/2  "SEA Torque"
  [Rthigh_cmd_trq] -> Add/1  "Motor Torque (before inefficiencies)"
  [Rthigh_cmd_trq] -> Mux10/3  "R_front_cmd (before inefficiencies)"
  Add/1 -> Mux10/2  "R_front_estimated (sum of forces)"
  [ddq4] -> Net Rotor Inertia1/1
  Net Rotor Inertia1/1 -> Mux10/4  "R_front_meas (from accel)"
  [Rshin_ctrl_trq] -> Mux11/1  "R_back_des"
  [RtauB] -> Gain3/1
  [R_rotor_stiction_back] -> Gain5/1
  Gain5/1 -> Add1/3  "gear stiction"
  Gain3/1 -> Add1/2  "SEA Torque"
  [Rshin_cmd_trq] -> Add1/1  "Motor Torque (before inefficiencies)"
  [Rshin_cmd_trq] -> Mux11/3  "R_back_cmd (before inefficiencies)"
  Add1/1 -> Mux11/2  "R_back_estimated (sum of forces)"
  [ddq2] -> Net Rotor Inertia/1
  Net Rotor Inertia/1 -> Mux11/4  "R_back_meas (from accel)"
  [Lthigh_ctrl_trq] -> Mux12/1  "L_front_des"
  [LtauF] -> Gain6/1
  [L_rotor_stiction_front] -> Gain8/1
  Gain8/1 -> Add2/3  "gear stiction"
  Gain6/1 -> Add2/2  "SEA Torque"
  [Lthigh_cmd_trq] -> Add2/1  "Motor Torque (before inefficiencies)"
  [Lthigh_cmd_trq] -> Mux12/3  "L_front_cmd (before inefficiencies)"
  Add2/1 -> Mux12/2  "L_front_estimated (sum of forces)"
  [ddq8] -> Net Rotor Inertia3/1
  Net Rotor Inertia3/1 -> Mux12/4  "L_front_meas (from accel)"
  [Lshin_ctrl_trq] -> Mux13/1  "L_back_des"
  [LtauB] -> Gain9/1
  [L_rotor_stiction_back] -> Gain11/1
  Gain11/1 -> Add3/3  "gear stiction"
  Gain9/1 -> Add3/2  "SEA Torque"
  [Lshin_cmd_trq] -> Add3/1  "Motor Torque (before inefficiencies)"
  [Lshin_cmd_trq] -> Mux13/3  "L_back_cmd (before inefficiencies)"
  Add3/1 -> Mux13/2  "L_back_estimated (sum of forces)"
  [ddq6] -> Net Rotor Inertia2/1
  Net Rotor Inertia2/1 -> Mux13/4  "L_back_meas (from accel)"
  Mux11/1 -> Net Torques on Rotor (after gearbox)/1
  Mux10/1 -> Net Torques on Rotor (after gearbox)/2
  Mux13/1 -> Net Torques on Rotor (after gearbox)/3
  Mux12/1 -> Net Torques on Rotor (after gearbox)/4
  [RFootCnt] -> Switch/2
  [ddq2] -> Net Rotor Inertia4/1
  Net Rotor Inertia4/1 -> Switch/3  "J * ddq_gear"
  [RtauB] -> Switch/1  "spring deflection"
  [RFootCnt] -> Switch1/2
  [ddq4] -> Net Rotor Inertia5/1
  Net Rotor Inertia5/1 -> Switch1/3  "J * ddq_gear"
  [RtauF] -> Switch1/1  "spring deflection"
  [LFootCnt] -> Switch2/2
  [ddq6] -> Net Rotor Inertia6/1
  Net Rotor Inertia6/1 -> Switch2/3  "J * ddq_gear"
  [LtauB] -> Switch2/1  "spring deflection"
  [LFootCnt] -> Switch3/2
  [ddq8] -> Net Rotor Inertia7/1
  Net Rotor Inertia7/1 -> Switch3/3  "J * ddq_gear"
  [LtauF] -> Switch3/1  "spring deflection"
  [LFootCnt] -> Mux14/2  "L Contact Detection"
  [RFootCnt] -> Mux14/1  "R Contact Detection"
  Mux5/1 -> Desired vs Measured Torques/1
  Mux4/1 -> Desired vs Measured Torques/2
  Mux7/1 -> Desired vs Measured Torques/3
  Mux6/1 -> Desired vs Measured Torques/4
  Mux14/1 -> Desired vs Measured Torques/5
  [RM12_after_stiction] -> Mux87/4  "RM12_after_friction"
  [RM23_after_stiction] -> Mux84/4  "RM23_after_friction"
  [LM12_after_stiction] -> Mux93/4  "LM12_after_friction"
  [LM23_after_stiction] -> Mux104/4  "LM23_after_friction"
  [Rshin_cmd_trq] -> Mux86/3  "RtauB_cmd"
  [ddq2] -> Net Rotor Inertia8/1
  Net Rotor Inertia8/1 -> Mux86/4  "RtauB_from_accel"
  [Rthigh_cmd_trq] -> Mux85/3  "RtauF_cmd"
  [ddq4] -> Net Rotor Inertia9/1
  Net Rotor Inertia9/1 -> Mux85/4  "RtauF_from_accel"
  [Lshin_ctrl_trq] -> Mux2/1  "LtauB_des"
  [RtauF] -> Mux1/2  "LtauF_sea"
  [LtauB] -> Mux2/2  "LtauB_sea"
  [Rthigh_ctrl_trq] -> Mux1/1  "LtauF_des"
  [Lshin_cmd_trq] -> Mux2/3  "LtauB_cmd"
  [ddq6] -> Net Rotor Inertia10/1
  Net Rotor Inertia10/1 -> Mux2/4  "LtauB_from_accel"
  [Lthigh_cmd_trq] -> Mux1/3  "LtauF_cmd"
  [ddq8] -> Net Rotor Inertia11/1
  Net Rotor Inertia11/1 -> Mux1/4  "LtauF_from_accel"
  Mux84/1 -> R Torques/1
  Mux87/1 -> R Torques/2
  Mux86/1 -> R Torques/3
  Mux85/1 -> R Torques/4
  [RFootCnt] -> R Torques/5  "R Contact Detection"
  Mux104/1 -> L Torques/1
  Mux93/1 -> L Torques/2
  Mux2/1 -> L Torques/3
  Mux1/1 -> L Torques/4
  [LFootCnt] -> L Torques/5  "L Contact Detection"
  [Rtau_pd_front] -> Mux15/2  "RtauF_pd"
  [Rtau_pd_back] -> Mux15/1  "RtauB_pd"
  [Ltau_pd_front] -> Mux15/4  "LtauF_pd"
  [Ltau_pd_back] -> Mux15/3  "LtauB_pd"
  [Rshin_cmd_trq] -> Mux3/1  "R_back_cmd"
  [Rthigh_cmd_trq] -> Mux3/2  "R_front_cmd"
  Mux3/1 -> "Cmd, PD, Scale, dTau, Stiction"/1
  [Lshin_cmd_trq] -> Mux3/3  "L_back_cmd"
  [Lthigh_cmd_trq] -> Mux3/4  "L_front_cmd"
  [R_scale_back] -> Mux8/1  "Rshin_scale"
  [R_scale_front] -> Mux8/2  "Rthigh_scale"
  [L_scale_back] -> Mux8/3  "Lshin_scale"
  [L_scale_front] -> Mux8/4  "Lthigh_scale"
  Mux8/1 -> "Cmd, PD, Scale, dTau, Stiction"/3
  [dRshin_des_trq] -> Mux9/1  "dTau_Rshin_des"
  [dRthigh_des_trq] -> Mux9/2  "dTau_Rthigh_des"
  [dLshin_des_trq] -> Mux9/3  "dTau_Lshin_des"
  [dLthigh_des_trq] -> Mux9/4  "dTau_Lthigh_des"
  Mux9/1 -> "Cmd, PD, Scale, dTau, Stiction"/4
  Mux15/1 -> "Cmd, PD, Scale, dTau, Stiction"/2
  [R_rotor_stiction_front] -> Gain4/1
  Gain4/1 -> Mux16/2  "(R Front) gear stiction"
  [R_rotor_stiction_back] -> Gain7/1
  Gain7/1 -> Mux16/1  "(R Back) gear stiction"
  [L_rotor_stiction_front] -> Gain10/1
  Gain10/1 -> Mux16/4  "(L Front) gear stiction"
  [L_rotor_stiction_back] -> Gain1/1
  Gain1/1 -> Mux16/3  "(L Back) gear stiction"
  Mux16/1 -> "Cmd, PD, Scale, dTau, Stiction"/5

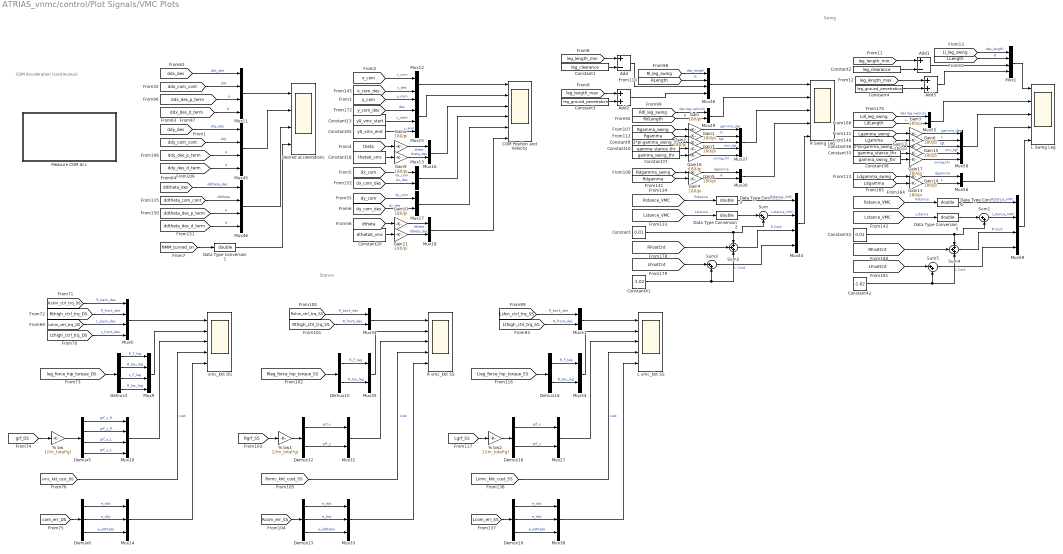
== system ATRIAS_vnmc/control/Plot Signals/VMC Plots ==
  note: COM Acceleration
      | (continuous)
  note: Stance
  note: Swing
  % bw : Gain  Gain=1/(m_total*g)
  % bw1 : Gain  Gain=1/(m_total*g)
  % bw2 : Gain  Gain=1/(m_total*g)
  Add : Sum  Inputs=+-
  Add1 : Sum  Inputs=+-
  Add2 : Sum
  Add3 : Sum
  COM Position and Velocity : Scope  NumInputPorts=6
      settings: ShowLegends=on  TimeRange=3.65  YMin=1.058~0.9~-0.5~-0.1~-0.3~-10  YMax=1.066~0.94~0.5~0.05~0~20  SaveName=ScopeData25
  Constant : Constant  Value=0.01
  Constant1 : Constant  Value=leg_clearance
  Constant10 : Constant  Value=gamma_stance_thr
  Constant13 : Constant  Value=y0_vmc_start
  Constant18 : Constant  Value=theta0_vmc
  Constant2 : Constant  Value=leg_clearance
  Constant20 : Constant  Value=dtheta0_vmc
  Constant3 : Constant  Value=leg_ground_penetration
  Constant32 : Constant  Value=0.01
  Constant33 : Constant  Value=gamma_stance_thr
  Constant36 : Constant  Value=2*pi-gamma_swing_thr
  Constant37 : Constant  Value=gamma_swing_thr
  Constant38 : Constant  Value=gamma_swing_thr
  Constant4 : Constant  Value=leg_ground_penetration
  Constant41 : Constant  Value=-1.02
  Constant42 : Constant  Value=-1.02
  Constant45 : Constant  Value=y0_vmc_end
  Constant9 : Constant  Value=2*pi-gamma_swing_thr
  Data Type Conversion{1..3,5..6} (5 alike) : DataTypeConversion  OutDataTypeStr=double
  Demux{10,12,16,18} (4 alike) : Demux  Outputs=2
  Demux13 : Demux  Outputs=3
  Demux19 : Demux  Outputs=3
  Demux3 : Demux
  Demux5 : Demux
  Demux6 : Demux  Outputs=3
  Desired accelerations : Scope  NumInputPorts=4
      settings: ShowLegends=on  YMin=-10~-10~-40~-5  YMax=5~15~40~5  SaveName=ScopeData50
  Gain{,1..17} (18 alike) : Gain  Gain=180/pi
  "L Swing Leg " : Scope  NumInputPorts=5
      settings: ShowLegends=on  TimeRange=1.035  YMin=0.5~-3~150~-200~0  YMax=1~4~210~150~1.2  SaveName=ScopeData54
  L vmc_kkt SS : Scope  NumInputPorts=5
      settings: ShowLegends=on  YMin=-1000~-500~0~0~-10  YMax=1000~1500~1000~100~5  SaveName=ScopeData53
  Measure COM Acc : Subsystem
  Mux{1,8..11,15,36,44..46,59} (11 alike) : Mux
  Mux{12..13,16..18,27,29..30,32,34..35,51,54..56} (15 alike) : Mux  Inputs=2
  Mux14 : Mux  Inputs=3
  Mux33 : Mux  Inputs=3
  Mux37 : Mux  Inputs=5
  Mux38 : Mux  Inputs=3
  Mux58 : Mux  Inputs=5
  R Swing Leg : Scope  NumInputPorts=5
      settings: ShowLegends=on  TimeRange=1.035  YMin=0.5~-3~150~-200~0  YMax=1~4~210~150~1.2  SaveName=ScopeData36
  R vmc_kkt SS : Scope  NumInputPorts=5
      settings: ShowLegends=on  YMin=-500~-500~-0.5~0~-30  YMax=500~1500~2.5~300~10  SaveName=ScopeData34
  Sum{,1,3,5} (4 alike) : Sum  Inputs=|++
  Sum2 : Sum  Inputs=+++
  Sum4 : Sum  Inputs=+++
  vmc_kkt DS : Scope  NumInputPorts=5
      settings: ShowLegends=on  YMin=-300~-200~-0.5~0~-0.1  YMax=200~600~1~500~0.4  SaveName=ScopeData26
  wires:
  [Rshin_ctrl_trq_DS] -> Mux8/1  "R_back_des"
  [Rthigh_ctrl_trq_DS] -> Mux8/2  "R_front_des"
  [Lshin_ctrl_trq_DS] -> Mux8/3  "L_back_des"
  [Lthigh_ctrl_trq_DS] -> Mux8/4  "L_front_des"
  Demux3/1 -> Mux9/1  "R_F_leg"
  Demux3/2 -> Mux9/2  "R_tau_leg"
  Demux3/3 -> Mux9/3  "L_F_leg"
  Demux3/4 -> Mux9/4  "R_tau_leg"
  Demux5/1 -> Mux10/1  "grf_x_R"
  Demux5/2 -> Mux10/2  "grf_y_R"
  Demux5/3 -> Mux10/3  "grf_x_L"
  Demux5/4 -> Mux10/4  "grf_y_L"
  Mux8/1 -> vmc_kkt DS/1
  Mux9/1 -> vmc_kkt DS/2
  Mux10/1 -> vmc_kkt DS/3
  Demux6/1 -> Mux14/1  "e_ddx"
  Demux6/2 -> Mux14/2  "e_ddy"
  Demux6/3 -> Mux14/3  "e_ddtheta"
  Mux14/1 -> vmc_kkt DS/5
  [x_com] -> Mux12/1  "x_com"
  [y_com] -> Mux15/1  "y_com"
  [theta] -> Gain8/1
  Mux12/1 -> COM Position and Velocity/1
  [dx_com] -> Mux13/1  "dx_com"
  [dy_com] -> Mux17/1  "dy_com"
  [dtheta] -> Gain10/1
  [ddy_des] -> Mux45/1  "ddy_des"
  [ddtheta_des] -> Mux46/1  "ddtheta_des"
  [ddx_des] -> Mux11/1  "ddx_des"
  [leg_force_hip_torque_DS] -> Demux3/1
  [grf_DS] -> % bw/1
  [com_err_DS] -> Demux6/1
  [vmc_kkt_cost_DS] -> vmc_kkt DS/4  "cost"
  [x_com_des] -> Mux12/2  "x_des"
  [dx_com_des] -> Mux13/2  "dx_des"
  Constant13/1 -> Mux15/3  "y_start"
  Constant18/1 -> Gain9/1
  [dy_com_des] -> Mux17/2  "dy_des"
  Constant20/1 -> Gain11/1
  Mux15/1 -> COM Position and Velocity/2
  Mux16/1 -> COM Position and Velocity/3
  Mux13/1 -> COM Position and Velocity/4
  Mux17/1 -> COM Position and Velocity/5
  Mux18/1 -> COM Position and Velocity/6
  [Rshin_ctrl_trq_SS] -> Mux34/1  "R_back_des"
  [Rthigh_ctrl_trq_SS] -> Mux34/2  "R_front_des"
  Demux10/1 -> Mux35/1  "R_F_leg"
  Demux10/2 -> Mux35/2  "R_tau_leg"
  Demux12/1 -> Mux32/1  "grf_x"
  Demux12/2 -> Mux32/2  "grf_y"
  Mux34/1 -> R vmc_kkt SS/1
  Mux35/1 -> R vmc_kkt SS/2
  Mux32/1 -> R vmc_kkt SS/3
  Demux13/1 -> Mux33/1  "e_ddx"
  Demux13/2 -> Mux33/2  "e_ddy"
  Demux13/3 -> Mux33/3  "e_ddtheta"
  Mux33/1 -> R vmc_kkt SS/5
  [Rleg_force_hip_torque_SS] -> Demux10/1
  [Rgrf_SS] -> % bw1/1
  [Rcom_err_SS] -> Demux13/1
  [Rvmc_kkt_cost_SS] -> R vmc_kkt SS/4  "cost"
  [Rl_leg_swing] -> Mux36/1  "des_length"
  [Rdgamma_swing] -> Gain4/1
  [Rgamma_swing] -> Gain/1
  [Rdl_leg_swing] -> Mux29/1  "des leg velocity"
  Gain/1 -> Mux37/1  "gamma_des"
  Gain4/1 -> Mux30/1  "dgamma"
  [RLength] -> Mux36/2  "R"
  Mux37/1 -> R Swing Leg/3
  [Rgamma] -> Gain1/1
  Gain1/1 -> Mux37/2  "R"
  Mux36/1 -> R Swing Leg/1
  [Rstance_VMC] -> Data Type Conversion3/1  "Rstance"
  [Lstance_VMC] -> Data Type Conversion2/1  "Lstance"
  Mux44/1 -> R Swing Leg/5
  [ddx_com_cont] -> Mux11/2  "ddx"
  [ddy_com_cont] -> Mux45/2  "ddy"
  [ddtheta_com_cont] -> Mux46/2  "ddtheta"
  Mux11/1 -> Desired accelerations/1
  Mux45/1 -> Desired accelerations/2
  Mux46/1 -> Desired accelerations/3
  [RdLength] -> Mux29/2  "R"
  Mux29/1 -> R Swing Leg/2
  [Rdgamma] -> Gain5/1
  Gain5/1 -> Mux30/2  "R"
  Mux30/1 -> R Swing Leg/4
  Constant/1 -> Sum/2, Sum2/1
  Sum/1 -> Mux44/2  "Lstance_VMC"
  Data Type Conversion2/1 -> Sum/1
  Data Type Conversion3/1 -> Mux44/1  "Rstance_VMC"
  Constant9/1 -> Gain2/1
  Constant10/1 -> Gain7/1
  Gain2/1 -> Mux37/3  "tgt"
  Gain7/1 -> Mux37/4  "min_tgt"
  Gain8/1 -> Mux16/1  "theta"
  Gain9/1 -> Mux16/2  "theta_des"
  Gain10/1 -> Mux18/1  "dtheta"
  Gain11/1 -> Mux18/2  "dtheta_des"
  % bw/1 -> Demux5/1
  % bw1/1 -> Demux12/1
  [ddx_des_p_term] -> Mux11/3  "p"
  [ddx_des_d_term] -> Mux11/4  "d"
  [ddy_des_p_term] -> Mux45/3  "p"
  [ddy_des_d_term] -> Mux45/4  "d"
  [ddtheta_des_p_term] -> Mux46/3  "p"
  [ddtheta_des_d_term] -> Mux46/4  "d"
  [Lshin_ctrl_trq_SS] -> Mux51/1  "R_back_des"
  [Lthigh_ctrl_trq_SS] -> Mux51/2  "R_front_des"
  Demux16/1 -> Mux54/1  "R_F_leg"
  Demux16/2 -> Mux54/2  "R_tau_leg"
  Demux18/1 -> Mux27/1  "grf_x"
  Demux18/2 -> Mux27/2  "grf_y"
  Mux51/1 -> L vmc_kkt SS/1
  Mux54/1 -> L vmc_kkt SS/2
  Mux27/1 -> L vmc_kkt SS/3
  Demux19/1 -> Mux38/1  "e_ddx"
  Demux19/2 -> Mux38/2  "e_ddy"
  Demux19/3 -> Mux38/3  "e_ddtheta"
  Mux38/1 -> L vmc_kkt SS/5
  [Lleg_force_hip_torque_SS] -> Demux16/1
  [Lgrf_SS] -> % bw2/1
  [Lcom_err_SS] -> Demux19/1
  [Lvmc_kkt_cost_SS] -> L vmc_kkt SS/4  "cost"
  % bw2/1 -> Demux18/1
  [Ldgamma_swing] -> Gain13/1
  [Lgamma_swing] -> Gain3/1
  [Ldl_leg_swing] -> Mux55/1  "des leg velocity"
  Gain3/1 -> Mux58/1  "gamma_des"
  Gain13/1 -> Mux56/1  "dgamma"
  Mux58/1 -> "L Swing Leg "/3
  [Lgamma] -> Gain6/1
  Gain6/1 -> Mux58/2  "L"
  [LdLength] -> Mux55/2  "L"
  Mux55/1 -> "L Swing Leg "/2
  [Ldgamma] -> Gain14/1
  Gain14/1 -> Mux56/2  "L"
  Mux56/1 -> "L Swing Leg "/4
  Constant36/1 -> Gain12/1
  Constant33/1 -> Gain15/1
  Gain12/1 -> Mux58/3  "tgt"
  Gain15/1 -> Mux58/4  "min_tgt"
  Constant37/1 -> Gain16/1
  Gain16/1 -> Mux37/5  "swing_thr"
  Constant38/1 -> Gain17/1
  Gain17/1 -> Mux58/5  "swing_thr"
  [RFootCnt] -> Sum2/2
  [LFootCnt] -> Sum3/1
  Constant41/1 -> Sum2/3, Sum3/2
  Sum2/1 -> Mux44/3  "R Cont"
  Sum3/1 -> Mux44/4  "L Cont"
  [Rstance_VMC] -> Data Type Conversion6/1  "Rstance"
  [Lstance_VMC] -> Data Type Conversion5/1  "Lstance"
  Mux59/1 -> "L Swing Leg "/5
  Constant32/1 -> Sum1/2, Sum4/1
  Sum1/1 -> Mux59/2  "Lstance_VMC"
  Data Type Conversion5/1 -> Sum1/1
  Data Type Conversion6/1 -> Mux59/1  "Rstance_VMC"
  [RFootCnt] -> Sum4/2
  [LFootCnt] -> Sum5/1
  Constant42/1 -> Sum4/3, Sum5/2
  Sum4/1 -> Mux59/3  "R Cont"
  Sum5/1 -> Mux59/4  "L Cont"
  Constant45/1 -> Mux15/4  "y_end"
  [y_com_des] -> Mux15/2  "des"
  [NMM_turned_on] -> Data Type Conversion1/1
  Data Type Conversion1/1 -> Desired accelerations/4
  [leg_length_min] -> Add/1
  Add/1 -> Mux36/3
  Constant1/1 -> Add/2
  [leg_length_max] -> Add2/1
  [Ll_leg_swing] -> Mux1/1  "des_length"
  [LLength] -> Mux1/2  "R"
  Mux1/1 -> "L Swing Leg "/1
  [leg_length_min] -> Add1/1
  Add1/1 -> Mux1/3
  Constant2/1 -> Add1/2
  Constant3/1 -> Add2/2
  Add2/1 -> Mux36/4
  [leg_length_max] -> Add3/1
  Constant4/1 -> Add3/2
  Add3/1 -> Mux1/4

== system ATRIAS_vnmc/control/Plot Signals/Virtual Angles ==
  Constant : Constant  Value=phi12_max
  Constant1 : Constant  Value=phi12_min
  Constant11 : Constant  Value=45*pi/180
  Constant3 : Constant  Value=phi23_max
  Constant4 : Constant  Value=phi23_min
  Gain{,1..14,16..20,22,26..28} (24 alike) : Gain  Gain=180/pi
  Gain15 : Gain  Gain=-180/pi
  "Leg Lengths, xTorso, dxTorso" : Scope  NumInputPorts=4
      settings: ShowLegends=on  TimeRange=0.4128245136433643  YMin=1~50~-5~-5  YMax=3.5~110~5~5  SaveName=ScopeData52
  Mux{1..7,81..83} (10 alike) : Mux  Inputs=2
  Mux27 : Mux
  Mux28 : Mux
  Mux32 : Mux
  Virtual Joint Angles : Scope  NumInputPorts=3
      settings: ShowLegends=on  TimeRange=0.8951752322126555  YMin=-50~100~0  YMax=50~250~180  SaveName=ScopeData29
  Virtual Joint Velocities : Scope  NumInputPorts=3
      settings: ShowLegends=on  TimeRange=0.8951752322126555  YMin=-30~-800~-1500  YMax=40~400~1000  SaveName=ScopeData51
  "k, alpha, dalpha" : Scope  NumInputPorts=4
      settings: ShowLegends=on  TimeRange=0.4128245136433643  YMin=1~85~80~-150  YMax=3~105~92~100
  wires:
  [Rphi12] -> Gain1/1
  Gain/1 -> Mux27/1  "Lphi12"
  Constant/1 -> Gain2/1
  Constant1/1 -> Gain3/1
  Mux27/1 -> Virtual Joint Angles/3
  [Rphi23] -> Gain5/1
  [Lphi23] -> Gain4/1
  Constant3/1 -> Gain6/1
  Constant4/1 -> Gain7/1
  Mux28/1 -> Virtual Joint Angles/2
  [Lphi12] -> Gain/1
  Gain1/1 -> Mux27/2  "Rphi12"
  Gain2/1 -> Mux27/3  "max"
  Gain3/1 -> Mux27/4  "max"
  Gain4/1 -> Mux28/1  "Lphi23"
  Gain5/1 -> Mux28/2  "Rphi23"
  Gain6/1 -> Mux28/3  "max"
  Gain7/1 -> Mux28/4  "min"
  Gain12/1 -> Mux32/1  "theta"
  [theta] -> Gain12/1
  Gain13/1 -> Mux32/2  "theta_tgt"
  [theta_tgt] -> Gain13/1
  Constant11/1 -> Gain15/1, Gain14/1
  Gain14/1 -> Mux32/3  "theta_max"
  Gain15/1 -> Mux32/4  "theta_min"
  Mux32/1 -> Virtual Joint Angles/1
  Gain9/1 -> Mux81/2  "Lalpha_tgt"
  Gain8/1 -> Mux81/1  "Lalpha"
  [Lalpha] -> Gain8/1
  [Lalpha_tgt] -> Gain9/1
  Gain11/1 -> Mux82/2  "Ralpha_tgt"
  Gain10/1 -> Mux82/1  "Ralpha"
  [Ralpha] -> Gain10/1
  [Ralpha_tgt] -> Gain11/1
  [xTorso] -> Mux83/1  "xTorso [m]"
  [yaw] -> Gain16/1  "yaw"
  [k_R] -> Mux1/1  "Jacobian Constant kR"
  [k_L] -> Mux1/2  "Jacobian Constant kL"
  Mux1/1 -> "k, alpha, dalpha"/1
  Mux81/1 -> "k, alpha, dalpha"/2
  Mux82/1 -> "k, alpha, dalpha"/3
  Gain16/1 -> Mux83/2  "yaw"
  [dxTorso] -> Mux2/1  "dxTorso [m]"
  [dyaw] -> Gain17/1  "dyaw"
  Gain17/1 -> Mux2/2  "dyaw"
  [Rdphi12] -> Gain19/1
  Gain18/1 -> Mux3/1  "Ldphi12"
  Mux3/1 -> Virtual Joint Velocities/3
  [Rdphi23] -> Gain27/1
  [Ldphi23] -> Gain26/1
  Mux4/1 -> Virtual Joint Velocities/2
  [Ldphi12] -> Gain18/1
  Gain19/1 -> Mux3/2  "Rdphi12"
  Gain26/1 -> Mux4/1  "Ldphi23"
  Gain27/1 -> Mux4/2  "Rdphi23"
  Gain20/1 -> Virtual Joint Velocities/1  "dtheta"
  [dtheta] -> Gain20/1
  Gain28/1 -> Mux7/1  "L dalpha"
  [Ldalpha] -> Gain28/1
  Gain22/1 -> Mux7/2  "R dalpha"
  [Rdalpha] -> Gain22/1
  [LLength] -> Mux5/1
  [RLength] -> Mux5/2
  [LdLength] -> Mux6/1
  [RdLength] -> Mux6/2
  Mux5/1 -> "Leg Lengths, xTorso, dxTorso"/1
  Mux6/1 -> "Leg Lengths, xTorso, dxTorso"/2
  Mux83/1 -> "Leg Lengths, xTorso, dxTorso"/3
  Mux2/1 -> "Leg Lengths, xTorso, dxTorso"/4
  Mux7/1 -> "k, alpha, dalpha"/4
